simulink model "IBSMC_f2"  (R2016b)
settings: Solver=VariableStepAuto  StartTime=0.0  StopTime=25  RelTol=1e-3
values from neighbouring files (symbols this model uses):
  a1 = 0.5*eye(3)    [cons2.m]
  a2 = 0.5*eye(3)    [cons2.m]
  j = diag([2.35e-3 2.35e-3 5.26e-2])    [cons2.m]
  k1 = 0.5*eye(3)    [cons2.m]
  k2 = 10*eye(3)    [cons2.m]
undefined symbols (not defined in the file or in its folder): q1, q2
settings Model: Creator=Ali  LastModifiedBy=Ali

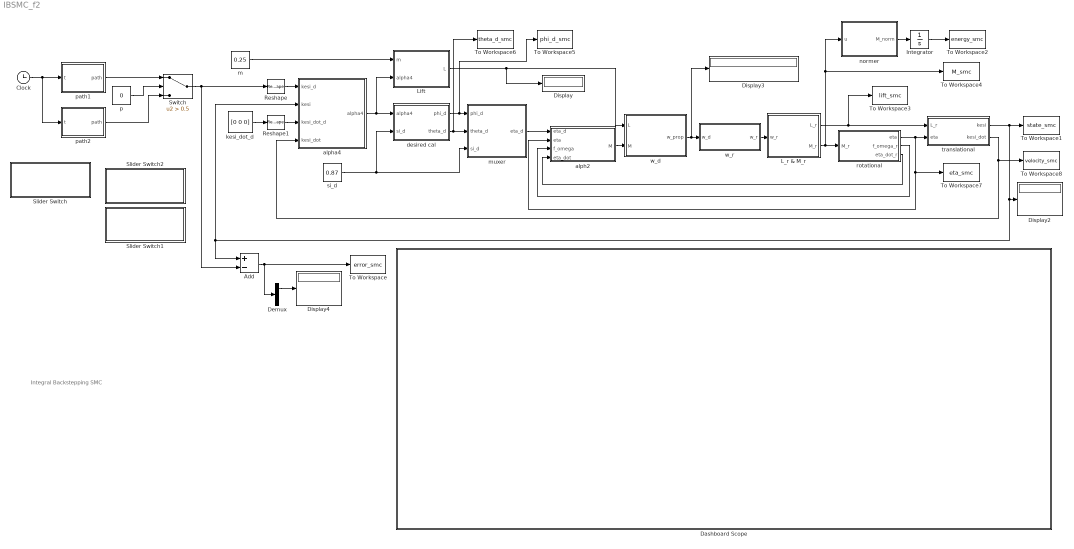
== system IBSMC_f2 ==
  note: Integral Backstepping SMC
  Add : Sum  Inputs=+-
  Clock : Clock
  Dashboard Scope : Subsystem  DialogController=hmiCreateDDGDialog  IsWebBlock=on  mask(MWDashboardBlock){webBlockId=683f2acd-1ab5-4fe6-a1c5-e24707c0b9b5, webBlockType=sdiscope, ShowInitialText=on, HMISrcModelName=IBSMC_f2}
      mask prompts: webBlockId "WebBlock Id"; webBlockType "WebBlock Type"; HMISrcModelName "Source Model"
      mask help: SimulinkHMI:dialogs:HMIScopeDialogDesc
      mask Help: helpview([docroot '/mapfiles/simulink.map'], 'hmi_scope')
      mask Display:
      | if strcmp(get_param(bdroot(gcb),'BlockDiagramType'), 'library')
      |     image([(matlabroot) '/toolbox/simulink/hmi/icons/DashboardScope.png']);
      | end
  Demux : Demux  Outputs=3
  Display{,2..4} (4 alike) : Display
  Integrator : Integrator
  L_r & M_r : MATLAB Function  TreatAsAtomicUnit=on
  Lift : MATLAB Function  TreatAsAtomicUnit=on
  Reshape : Reshape  OutputDimensionality=Column vector (2-D)
  Reshape1 : Reshape  OutputDimensionality=Column vector (2-D)
  Slider Switch : Subsystem  DialogController=hmiCreateDDGDialog  IsWebBlock=on  mask(MWDashboardBlock){webBlockId=6a64296e-d80f-4a95-af95-452b2e7ac7b4, webBlockType=sliderswitch, ShowInLibBrowser=on, ShowInitialText=on, HMISrcModelName=IBSMC_f2}
      mask prompts: webBlockId "WebBlock Id"; webBlockType "WebBlock Type"; HMISrcModelName "Source Model"
      mask help: SimulinkHMI:dialogs:SwitchDialogDesc
      mask Help: helpview([docroot '/mapfiles/simulink.map'], 'hmi_slider_switch')
      mask Display:
      | if strcmp(get_param(bdroot(gcb),'BlockDiagramType'), 'library')
      |     image([(matlabroot) '/toolbox/simulink/hmi/icons/SliderSwitch.png']);
      | end
  Slider Switch1 : Subsystem  DialogController=hmiCreateDDGDialog  IsWebBlock=on  mask(MWDashboardBlock){webBlockId=af26f90a-f7c1-418a-b158-ebb9c4ca13f4, webBlockType=sliderswitch, ShowInLibBrowser=on, ShowInitialText=on, HMISrcModelName=IBSMC_f2}
      mask prompts: webBlockId "WebBlock Id"; webBlockType "WebBlock Type"; HMISrcModelName "Source Model"
      mask help: SimulinkHMI:dialogs:SwitchDialogDesc
      mask Help: helpview([docroot '/mapfiles/simulink.map'], 'hmi_slider_switch')
      mask Display:
      | if strcmp(get_param(bdroot(gcb),'BlockDiagramType'), 'library')
      |     image([(matlabroot) '/toolbox/simulink/hmi/icons/SliderSwitch.png']);
      | end
  Slider Switch2 : Subsystem  DialogController=hmiCreateDDGDialog  IsWebBlock=on  mask(MWDashboardBlock){webBlockId=08faa15c-f6c0-4120-bff0-043c57088010, webBlockType=sliderswitch, ShowInLibBrowser=on, ShowInitialText=on, HMISrcModelName=IBSMC_f2}
      mask prompts: webBlockId "WebBlock Id"; webBlockType "WebBlock Type"; HMISrcModelName "Source Model"
      mask help: SimulinkHMI:dialogs:SwitchDialogDesc
      mask Help: helpview([docroot '/mapfiles/simulink.map'], 'hmi_slider_switch')
      mask Display:
      | if strcmp(get_param(bdroot(gcb),'BlockDiagramType'), 'library')
      |     image([(matlabroot) '/toolbox/simulink/hmi/icons/SliderSwitch.png']);
      | end
  Switch : Switch  Criteria=u2 > Threshold  Threshold=0.5
  To Workspace : ToWorkspace  VariableName=error_smc  SampleTime=-1
  To Workspace1 : ToWorkspace  VariableName=state_smc  SampleTime=-1
  To Workspace2 : ToWorkspace  VariableName=energy_smc  SampleTime=-1
  To Workspace3 : ToWorkspace  VariableName=lift_smc  SampleTime=-1
  To Workspace4 : ToWorkspace  VariableName=M_smc  SampleTime=-1
  To Workspace5 : ToWorkspace  VariableName=phi_d_smc  SampleTime=-1
  To Workspace6 : ToWorkspace  VariableName=theta_d_smc  SampleTime=-1
  To Workspace7 : ToWorkspace  VariableName=eta_smc  SampleTime=-1
  To Workspace8 : ToWorkspace  VariableName=velocity_smc  SampleTime=-1
  alph2 : Subsystem
  alpha4 : Subsystem
  desired cal : MATLAB Function  TreatAsAtomicUnit=on
  kesi_dot_d : Constant  Value=[0 0 0]
  m : Constant  Value=0.25
  muxer : MATLAB Function  TreatAsAtomicUnit=on
  normer : MATLAB Function  TreatAsAtomicUnit=on
  p : Constant  Value=0
  path1 : MATLAB Function  TreatAsAtomicUnit=on
  path2 : MATLAB Function  TreatAsAtomicUnit=on
  rotational : Subsystem
  si_d : Constant  Value=0.87
  translational : Subsystem
  w_d : MATLAB Function  TreatAsAtomicUnit=on
  w_r : Subsystem
  wires:
  si_d/1 -> desired cal/2(si_d), muxer/3(si_d)
  desired cal/1(phi_d) -> To Workspace5/1, muxer/1(phi_d)
  desired cal/2(theta_d) -> To Workspace6/1, muxer/2(theta_d)
  muxer/1(eta_d) -> alph2/1(eta_d)
  alpha4/1(alpha4) -> desired cal/1(alpha4), Lift/2(alpha4)
  m/1 -> Lift/1(m)
  alph2/1(M) -> w_d/2(M)
  Lift/1(L) -> Display/1, w_d/1(L)
  w_d/1(w_prop) -> Display3/1, w_r/1(w_d)
  w_r/1(w_r) -> L_r & M_r/1(w_r)
  L_r & M_r/2(M_r) -> To Workspace4/1, normer/1(u), rotational/1(M_r)
  rotational/2(f_omega_r) -> alph2/3(f_omega)
  rotational/1(eta) -> alph2/2(eta), To Workspace7/1, translational/2(eta)
  translational/1(kesi) -> To Workspace1/1, Display2/1, Add/1, alpha4/2(kesi)
  Reshape/1 -> alpha4/1(kesi_d)
  Reshape1/1 -> alpha4/3(kesi_dot_d)
  kesi_dot_d/1 -> Reshape1/1
  translational/2(kesi_dot) -> To Workspace8/1, alpha4/4(kesi_dot)
  rotational/3(eta_dot_r) -> alph2/4(eta_dot)
  Clock/1 -> path2/1(t), path1/1(t)
  path1/1(path) -> Switch/1
  path2/1(path) -> Switch/3
  p/1 -> Switch/2
  Switch/1 -> Add/2, Reshape/1
  Demux/1 -> Display4/1
  Add/1 -> To Workspace/1, Demux/1
  L_r & M_r/1(L_r) -> To Workspace3/1, translational/1(L_r)
  normer/1(M_norm) -> Integrator/1
  Integrator/1 -> To Workspace2/1

== system IBSMC_f2/Dashboard Scope ==

== system IBSMC_f2/Slider Switch ==

== system IBSMC_f2/Slider Switch1 ==

== system IBSMC_f2/Slider Switch2 ==

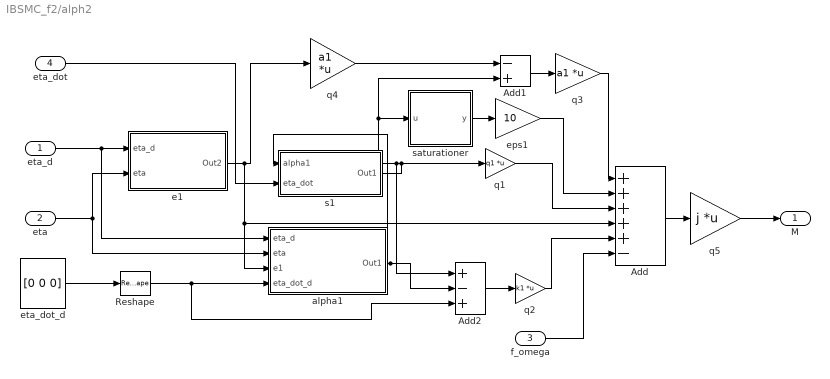
== system IBSMC_f2/alph2 ==
  eta_d : Inport
  eta : Inport  Port=2
  f_omega : Inport  Port=3
  eta_dot : Inport  Port=4
  Add : Sum  Inputs=+++++-
  Add1 : Sum  Inputs=-+
  Add2 : Sum  Inputs=+-+
  Reshape : Reshape  OutputDimensionality=Column vector (2-D)
  alpha1 : Subsystem
  e1 : Subsystem
  eps1 : Gain  Gain=10
  eta_dot_d : Constant  Value=[0 0 0]
  q1 : Gain  Gain=q1  Multiplication=Matrix(K*u)
  q2 : Gain  Gain=k1  Multiplication=Matrix(K*u)
  q3 : Gain  Gain=a1  Multiplication=Matrix(K*u)
  q4 : Gain  Gain=a1  Multiplication=Matrix(K*u)
  q5 : Gain  Gain=j  Multiplication=Matrix(K*u)
  s1 : Subsystem
  saturationer : MATLAB Function  TreatAsAtomicUnit=on
  M : Outport
  wires:
  eta_d/1 -> alpha1/1(eta_d), e1/1(eta_d)
  e1/1(Out2) -> q4/1, alpha1/3(e1), Add/4
  eta_dot_d/1 -> Reshape/1
  saturationer/1(y) -> eps1/1
  s1/1(Out1) -> saturationer/1(u), Add1/2, Add2/1, q1/1
  q5/1 -> M/1
  q1/1 -> Add/3
  eps1/1 -> Add/2
  f_omega/1 -> Add/6
  alpha1/1(Out1) -> s1/1(alpha1), Add2/2
  Add2/1 -> q2/1
  q2/1 -> Add/5
  q3/1 -> Add/1
  Add1/1 -> q3/1
  eta/1 -> e1/2(eta), alpha1/2(eta)
  Add/1 -> q5/1
  Reshape/1 -> Add2/3, alpha1/4(eta_dot_d)
  q4/1 -> Add1/1
  eta_dot/1 -> s1/2(eta_dot)

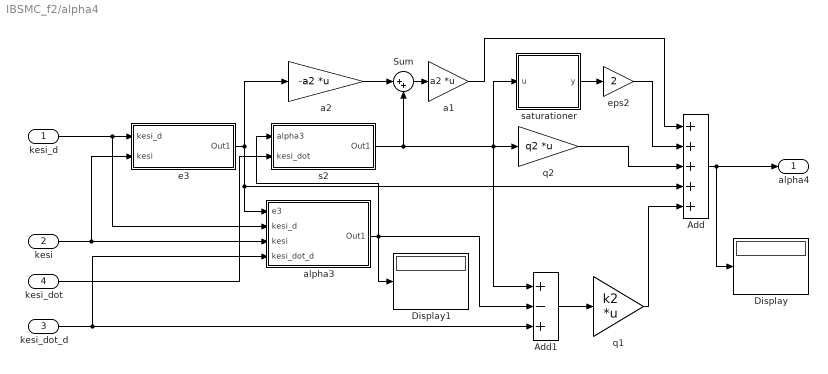
== system IBSMC_f2/alpha4 ==
  kesi_d : Inport
  kesi : Inport  Port=2
  kesi_dot_d : Inport  Port=3
  kesi_dot : Inport  Port=4
  Add : Sum  Inputs=+++++
  Add1 : Sum  Inputs=+-+
  Display : Display
  Display1 : Display
  Sum : Sum  Inputs=|++
  a1 : Gain  Gain=a2  Multiplication=Matrix(K*u)
  a2 : Gain  Gain=-a2  Multiplication=Matrix(K*u)
  alpha3 : Subsystem
  e3 : Subsystem
  eps2 : Gain  Gain=2
  q1 : Gain  Gain=k2  Multiplication=Matrix(K*u)
  q2 : Gain  Gain=q2  Multiplication=Matrix(K*u)
  s2 : Subsystem
  saturationer : MATLAB Function  TreatAsAtomicUnit=on
  alpha4 : Outport
  wires:
  saturationer/1(y) -> eps2/1
  q2/1 -> Add/3
  alpha3/1(Out1) -> Display1/1, s2/1(alpha3), Add1/2
  kesi/1 -> e3/2(kesi), alpha3/3(kesi)
  s2/1(Out1) -> Add1/1, q2/1, saturationer/1(u), Sum/2
  e3/1(Out1) -> alpha3/1(e3), Add/4, a2/1
  kesi_dot_d/1 -> alpha3/4(kesi_dot_d), Add1/3
  kesi_d/1 -> e3/1(kesi_d), alpha3/2(kesi_d)
  a2/1 -> Sum/1
  Sum/1 -> a1/1
  Add/1 -> alpha4/1, Display/1
  a1/1 -> Add/1
  Add1/1 -> q1/1
  q1/1 -> Add/5
  eps2/1 -> Add/2
  kesi_dot/1 -> s2/2(kesi_dot)

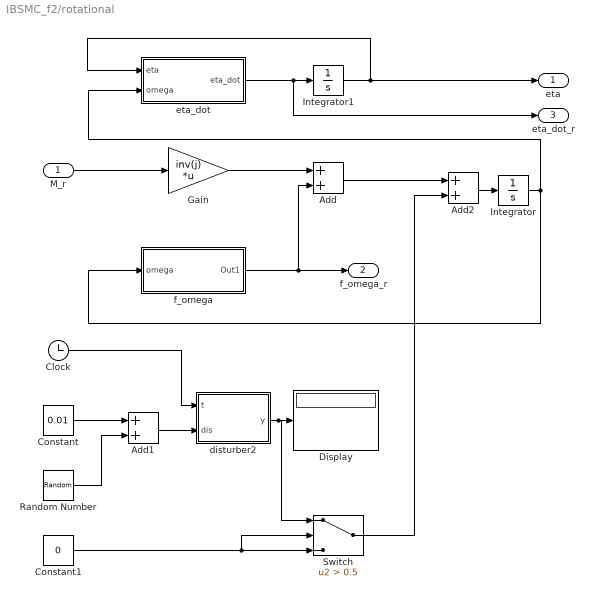
== system IBSMC_f2/rotational ==
  M_r : Inport
  Add : Sum
  Add1 : Sum
  Add2 : Sum
  Clock : Clock
  Constant : Constant  Value=0.01
  Constant1 : Constant  Value=0
  Display : Display
  Gain : Gain  Gain=inv(j)  Multiplication=Matrix(K*u)
  Integrator : Integrator
  Integrator1 : Integrator
  Random Number : RandomNumber  Variance=0.005  SampleTime=0.1
  Switch : Switch  Criteria=u2 > Threshold  Threshold=0.5
  disturber2 : MATLAB Function  TreatAsAtomicUnit=on
  eta_dot : Subsystem
  f_omega : Subsystem
  eta : Outport
  f_omega_r : Outport  Port=2
  eta_dot_r : Outport  Port=3
  wires:
  M_r/1 -> Gain/1
  Gain/1 -> Add/1
  f_omega/1(Out1) -> Add/2, f_omega_r/1
  Integrator/1 -> eta_dot/2(omega), f_omega/1(omega)
  eta_dot/1(eta_dot) -> eta_dot_r/1, Integrator1/1
  Integrator1/1 -> eta/1, eta_dot/1(eta)
  Constant/1 -> Add1/1
  Random Number/1 -> Add1/2
  Add1/1 -> disturber2/2(dis)
  Clock/1 -> disturber2/1(t)
  disturber2/1(y) -> Switch/1, Display/1
  Add/1 -> Add2/1
  Add2/1 -> Integrator/1
  Constant1/1 -> Switch/2, Switch/3
  Switch/1 -> Add2/2

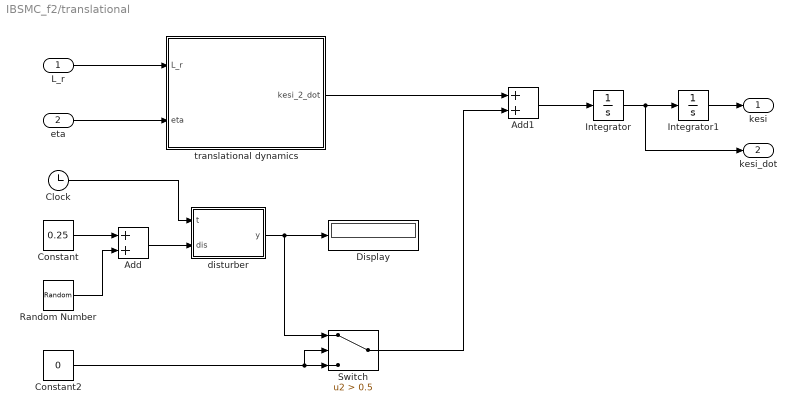
== system IBSMC_f2/translational ==
  L_r : Inport
  eta : Inport  Port=2
  Add : Sum
  Add1 : Sum
  Clock : Clock
  Constant : Constant  Value=0.25
  Constant2 : Constant  Value=0
  Display : Display
  Integrator : Integrator
  Integrator1 : Integrator
  Random Number : RandomNumber  Variance=0.01  SampleTime=0.1
  Switch : Switch  Criteria=u2 > Threshold  Threshold=0.5
  disturber : MATLAB Function  TreatAsAtomicUnit=on
  translational dynamics : MATLAB Function  TreatAsAtomicUnit=on
  kesi : Outport
  kesi_dot : Outport  Port=2
  wires:
  L_r/1 -> translational dynamics/1(L_r)
  eta/1 -> translational dynamics/2(eta)
  Integrator/1 -> Integrator1/1, kesi_dot/1
  Integrator1/1 -> kesi/1
  translational dynamics/1(kesi_2_dot) -> Add1/1
  Add1/1 -> Integrator/1
  Constant/1 -> Add/1
  Random Number/1 -> Add/2
  Add/1 -> disturber/2(dis)
  Clock/1 -> disturber/1(t)
  disturber/1(y) -> Display/1, Switch/1
  Constant2/1 -> Switch/2, Switch/3
  Switch/1 -> Add1/2

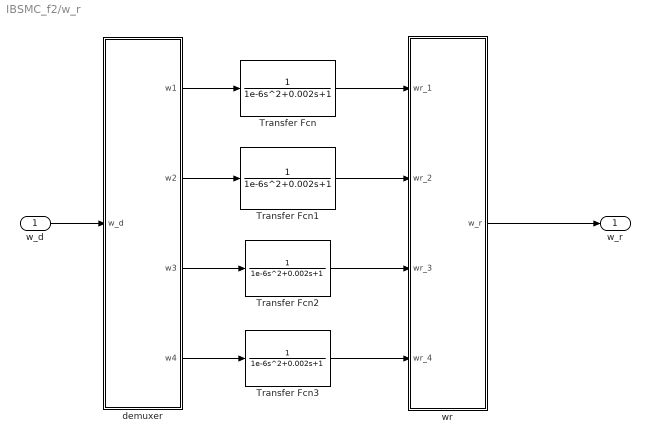
== system IBSMC_f2/w_r ==
  w_d : Inport
  Transfer Fcn{,1..3} (4 alike) : TransferFcn  Denominator=[1e-6 0.002 1]
  demuxer : MATLAB Function  TreatAsAtomicUnit=on
  wr : MATLAB Function  TreatAsAtomicUnit=on
  w_r : Outport
  wires:
  w_d/1 -> demuxer/1(w_d)
  wr/1(w_r) -> w_r/1
  demuxer/1(w1) -> Transfer Fcn/1
  demuxer/2(w2) -> Transfer Fcn1/1
  demuxer/3(w3) -> Transfer Fcn2/1
  demuxer/4(w4) -> Transfer Fcn3/1
  Transfer Fcn/1 -> wr/1(wr_1)
  Transfer Fcn1/1 -> wr/2(wr_2)
  Transfer Fcn2/1 -> wr/3(wr_3)
  Transfer Fcn3/1 -> wr/4(wr_4)

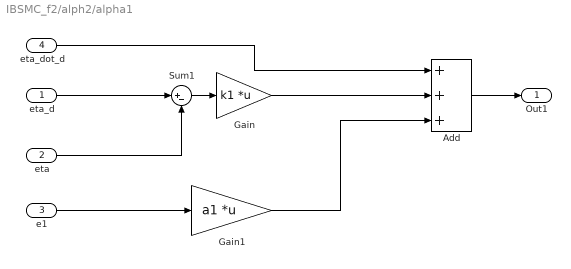
== system IBSMC_f2/alph2/alpha1 ==
  eta_d : Inport
  eta : Inport  Port=2
  e1 : Inport  Port=3
  eta_dot_d : Inport  Port=4
  Add : Sum  Inputs=+++
  Gain : Gain  Gain=k1  Multiplication=Matrix(K*u)
  Gain1 : Gain  Gain=a1  Multiplication=Matrix(K*u)
  Sum1 : Sum  Inputs=|+-
  Out1 : Outport
  wires:
  Add/1 -> Out1/1
  Sum1/1 -> Gain/1
  eta/1 -> Sum1/2
  eta_d/1 -> Sum1/1
  Gain/1 -> Add/2
  eta_dot_d/1 -> Add/1
  e1/1 -> Gain1/1
  Gain1/1 -> Add/3

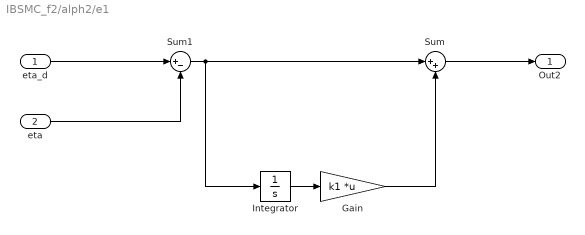
== system IBSMC_f2/alph2/e1 ==
  eta_d : Inport
  eta : Inport  Port=2
  Gain : Gain  Gain=k1  Multiplication=Matrix(K*u)
  Integrator : Integrator
  Sum : Sum  Inputs=|++
  Sum1 : Sum  Inputs=|+-
  Out2 : Outport
  wires:
  eta_d/1 -> Sum1/1
  eta/1 -> Sum1/2
  Sum1/1 -> Integrator/1, Sum/1
  Sum/1 -> Out2/1
  Gain/1 -> Sum/2
  Integrator/1 -> Gain/1

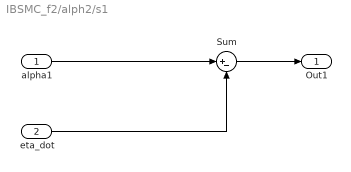
== system IBSMC_f2/alph2/s1 ==
  alpha1 : Inport
  eta_dot : Inport  Port=2
  Sum : Sum  Inputs=|+-
  Out1 : Outport
  wires:
  Sum/1 -> Out1/1
  alpha1/1 -> Sum/1
  eta_dot/1 -> Sum/2

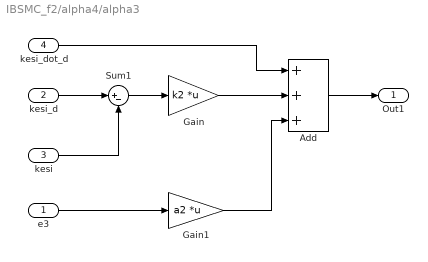
== system IBSMC_f2/alpha4/alpha3 ==
  e3 : Inport
  kesi_d : Inport  Port=2
  kesi : Inport  Port=3
  kesi_dot_d : Inport  Port=4
  Add : Sum  Inputs=+++
  Gain : Gain  Gain=k2  Multiplication=Matrix(K*u)
  Gain1 : Gain  Gain=a2  Multiplication=Matrix(K*u)
  Sum1 : Sum  Inputs=|+-
  Out1 : Outport
  wires:
  Add/1 -> Out1/1
  Sum1/1 -> Gain/1
  kesi/1 -> Sum1/2
  kesi_d/1 -> Sum1/1
  Gain/1 -> Add/2
  kesi_dot_d/1 -> Add/1
  e3/1 -> Gain1/1
  Gain1/1 -> Add/3

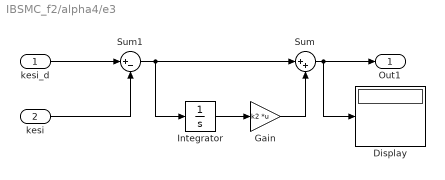
== system IBSMC_f2/alpha4/e3 ==
  kesi_d : Inport
  kesi : Inport  Port=2
  Display : Display
  Gain : Gain  Gain=k2  Multiplication=Matrix(K*u)
  Integrator : Integrator
  Sum : Sum  Inputs=|++
  Sum1 : Sum  Inputs=|+-
  Out1 : Outport
  wires:
  kesi_d/1 -> Sum1/1
  kesi/1 -> Sum1/2
  Sum1/1 -> Integrator/1, Sum/1
  Integrator/1 -> Gain/1
  Gain/1 -> Sum/2
  Sum/1 -> Out1/1, Display/1

== system IBSMC_f2/alpha4/s2 ==
  alpha3 : Inport
  kesi_dot : Inport  Port=2
  Sum : Sum  Inputs=|+-
  Out1 : Outport
  wires:
  Sum/1 -> Out1/1
  alpha3/1 -> Sum/1
  kesi_dot/1 -> Sum/2

== system IBSMC_f2/rotational/eta_dot ==
  eta : Inport
  omega : Inport  Port=2
  eta_dot_cal : MATLAB Function  TreatAsAtomicUnit=on
  eta_dot : Outport
  wires:
  eta_dot_cal/1(eta_dot) -> eta_dot/1
  eta/1 -> eta_dot_cal/1(eta)
  omega/1 -> eta_dot_cal/2(omega)

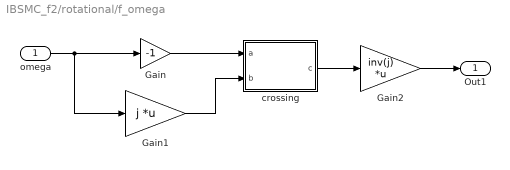
== system IBSMC_f2/rotational/f_omega ==
  omega : Inport
  Gain : Gain  Gain=-1
  Gain1 : Gain  Gain=j  Multiplication=Matrix(K*u)
  Gain2 : Gain  Gain=inv(j)  Multiplication=Matrix(K*u)
  crossing : MATLAB Function  TreatAsAtomicUnit=on
  Out1 : Outport
  wires:
  omega/1 -> Gain1/1, Gain/1
  Gain/1 -> crossing/1(a)
  Gain1/1 -> crossing/2(b)
  crossing/1(c) -> Gain2/1
  Gain2/1 -> Out1/1

== matlab function IBSMC_f2/desired cal ==
  data: alpha4 input; phi_d output; theta_d output; si_d input
function [phi_d,theta_d] = fcn(alpha4,si_d)
g=9.81;
phi_d=asin((alpha4(1)*sin(si_d)-alpha4(2)*cos(si_d))/sqrt(alpha4(1)^2+alpha4(2)^2+(alpha4(3)+g)^2));
theta_d = atan((alpha4(1)*cos(si_d)+alpha4(2)*sin(si_d))/(alpha4(3)+g));

== matlab function IBSMC_f2/Lift ==
  data: m input; alpha4 input; L output
function L = fcn(m,alpha4)
g=9.81;
L = sqrt(m^2*(alpha4(1)^2+alpha4(2)^2+(alpha4(3)+g)^2));

== matlab function IBSMC_f2/muxer ==
  data: phi_d input; eta_d output; theta_d input; si_d input
function eta_d = fcn(phi_d,theta_d,si_d)
eta_d = [phi_d;theta_d;si_d];

== matlab function IBSMC_f2/w_d ==
  data: L input; w_prop output; M input
function w_prop = fcn(L,M)
w_prop=zeros(4,1);
b=6.13e-5;d=0.2;kd=2.5e-6;
co=[b b b b;0 -d*b 0 d*b;-d*b 0 d*b 0;kd -kd kd -kd];
w_prop=inv(co)*[L;M];

== matlab function IBSMC_f2/w_r/demuxer ==
  data: w_d input; w1 output; w2 output; w3 output; w4 output
function [w1,w2,w3,w4]= fcn(w_d)
w1=w_d(1);
w2=w_d(2);
w3=w_d(3);
w4=w_d(4);

== matlab function IBSMC_f2/w_r/wr ==
  data: wr_1 input; w_r output; wr_2 input; wr_3 input; wr_4 input
function w_r = fcn(wr_1,wr_2,wr_3,wr_4)
w_r =[wr_1;wr_2;wr_3;wr_4];

== matlab function IBSMC_f2/L_r & M_r ==
  data: w_r input; L_r output; M_r output
function [L_r,M_r]= fcn(w_r)
b=6.13e-5;d=0.2;kd=2.5e-6;
co=[b b b b;0 -d*b 0 d*b;-d*b 0 d*b 0;kd -kd kd -kd];
ML=co*w_r;
L_r=ML(1);
M_r=ML(2:4);

== matlab function IBSMC_f2/rotational/eta_dot/eta_dot_cal ==
  data: eta input; eta_dot output; omega input
function eta_dot = fcn(eta,omega)
eta_dot=zeros(3,1);
phi=eta(1);
theta=eta(2);
w=[1 sin(phi)*tan(theta) cos(phi)*tan(theta);0 cos(phi) -sin(phi);0 sin(phi)/cos(theta) cos(phi)/cos(theta)];
eta_dot = w*omega;

== matlab function IBSMC_f2/translational/translational dynamics ==
  data: L_r input; kesi_2_dot output; eta input
function kesi_2_dot = fcn(L_r,eta)
kesi_2_dot=zeros(3,1);
m=0.25;g=9.81;
r_be=[cos(eta(3))*cos(eta(2)) cos(eta(2))*sin(eta(3)) -sin(eta(2));cos(eta(3))*sin(eta(1))*sin(eta(2))-cos(eta(1))*sin(eta(3)) cos(eta(1))*cos(eta(3))+sin(eta(1))*sin(eta(3))*sin(eta(2)) cos(eta(2))*sin(eta(1));sin(eta(1))*sin(eta(3))+cos(eta(1))*cos(eta(3))*sin(eta(2)) cos(eta(1))*sin(eta(3))*sin(eta(2))-cos(eta(3))*sin(eta(1)) cos(eta(1))*cos(eta(2))];
r_eb=r_be';
kesi_2_dot =r_eb*[0;0;L_r/m]+[0;0;-g];

== matlab function IBSMC_f2/alpha4/saturationer ==
  data: u input; y output
function y = fcn(u)
y=min(max(u*0.04,-[1;1;1]),[1;1;1]);

== matlab function IBSMC_f2/alph2/saturationer ==
  data: u input; y output
function y = fcn(u)
y=min(max(u*0.04,-[1;1;1]),[1;1;1]);

== matlab function IBSMC_f2/path2 ==
  data: t input; path output
function path= fcn(t)
path=zeros(3,1);
if t<=10
    x=5*t/10;
    y=4*t/10;
    z=3*t/10;
elseif 10<t & t<=15
     x=5;
    y=4;
    z=3;   
else
    x=0.5*(t-5);
    y=-0.4*t+10;
    z=-0.3*t+7.5;
end
path=[x;y;z];

== matlab function IBSMC_f2/translational/disturber ==
  data: t input; y output; dis input
function y = fcn(t,dis)
m=0.25;
if t>=50 & t<=60
    y=dis/m;
else
    y=0;
end

== matlab function IBSMC_f2/rotational/disturber2 ==
  data: t input; y output; dis input
function y = fcn(t,dis)
y=zeros(3,1);
if t>=150 & t<=160
    j=diag([2.35e-3 2.35e-3 5.26e-2]);
    y=inv(j)*dis*ones(3,1);
else
    y=zeros(3,1);
end

== matlab function IBSMC_f2/rotational/f_omega/crossing ==
  data: a input; c output; b input
function  c = fcn(a,b)
c=zeros(3,1);
c= cross(a,b);

== matlab function IBSMC_f2/path1 ==
  data: t input; path output
function path= fcn(t)
path=zeros(3,1);
x=5*cos(0.1*t)+5;
y=5*sin(0.1*t)+5;
z=0.3*t;
path=[x;y;z];

== matlab function IBSMC_f2/normer ==
  data: u input; M_norm output
function M_norm = fcn(u)
M_norm=sqrt(u(1)^2+u(2)^2+u(3)^2);
